simulink model "Model_RB_APF_WF_VO"  (R2024b)
settings: Solver=FixedStepAuto  StartTime=0.0  StopTime=120  FixedStep=UAVSampleTime  RelTol=1e-3
undefined symbols (not defined in the file): DroneMass, Gravity, Horizontal_Limits, Horizontal_Res, kD_pos, kD_vel, kI_pos, kI_vel, kP_pos, kP_vel, Lidar, MaxRange, N_filter, TopSpeed, UAV, Vertical_Limits, Vertical_Res, Waypoints
libraries: slpidlib x6, uavsimlib x4, robotcorelib x1, uavalgslib x1
(part 2 of 2)

== matlab function Model_RB_APF_WF_VO/WF/WFVectors ==
  data: flight_mode input; cloud input; radial_vec output; lateral_vec output; virtuals input; virtualCount input; pos input
function [radial_vec, lateral_vec] = WF(flight_mode, cloud, virtuals, virtualCount, pos)

% Parameters
comfort_zone = 2;
lateral_scaler = 0.5;
radial_scaler = 0.8;

% Initializations
n_points = size(cloud,1);
d_min = inf;                    % initialize with very large number
r_min = zeros(3,1);             % closest-point vector (radial)

% Loop through lidar points for closest point
for i = 1:n_points
    % Per particular pixel/ray

    r = -cloud(i,:).';         % 3x1 vector of distance 
    D = norm(r);               % scalar distance

    % check if this is the closest so far
    if D < d_min
        d_min = D;
        r_min = r;
    end
end

% Loop through VOs for closest point
for i = 1:virtualCount
    r = -(virtuals(i,1:3).' - pos);
    D = norm(r);
    % check if this is the closest so far
    if D < d_min
        d_min = D;
        r_min = r;
    end
end

% Radial
radial_dir = r_min / d_min;             % unit vector
radial_dif = (comfort_zone - d_min);
radial_vec = radial_dir*radial_dif*radial_scaler;

% Lateral
if flight_mode == 2
    rotation = -pi/2;   % Go Left
else
    rotation = pi/2;    % Go right
end

lateral_dir = axang2rotm([0 0 1 rotation])*radial_dir;  % this is rotating about z axis, not exactly orthogonal to raidal_vec
lateral_vec = lateral_dir*lateral_scaler;

== matlab function Model_RB_APF_WF_VO/APF/APF_Limiter1 ==
  data: del_U input; gradientCapped output
function gradientCapped = limiter(del_U)

maximum = 5;

mag = norm(del_U);

if mag > maximum
    gradientCapped = maximum*(del_U/mag);
else
    gradientCapped = del_U;
end
